simulink model "LQR_control"  (R2025b)
settings: Solver=VariableStepAuto  StartTime=0.0  StopTime=10.0  RelTol=1e-3
values from neighbouring files (symbols this model uses):
  A_Mat = [ 0     1    0     0 ... (first row only)    [LQR_code.m]
  B_Mat = [ 0 ... (first row only)    [LQR_code.m]
  C_Mat = [ 1  0    0   0 ... (first row only)    [LQR_code.m]
  K = lqr(A_Mat, B_Mat, Q, R)    [LQR_code.m]
settings Model: Creator=Mahmoud Essam  LastModifiedBy=Mahmoud Essam

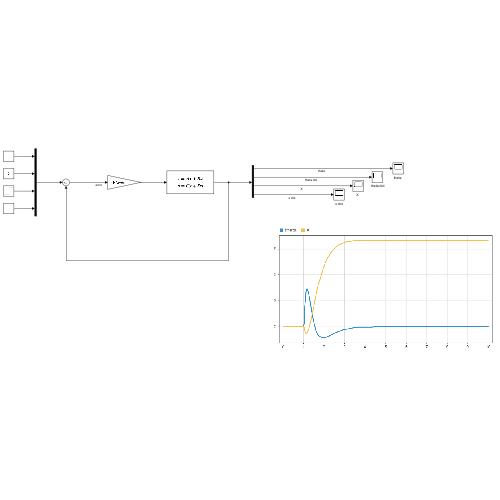
[thumbnail: Simulink's stored preview of the top-level diagram]
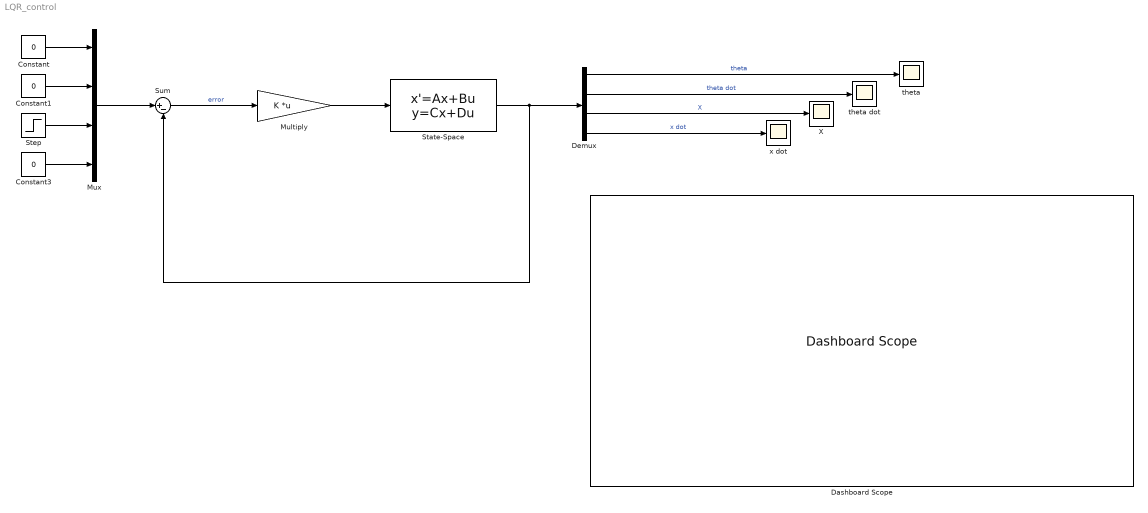
== system LQR_control ==
  " theta dot" : Scope
      settings: ActiveDisplayYMinimum=-22.999413149940512  ActiveDisplayYMaximum=55.548140907039681
  Constant : Constant  Value=0
  Constant1 : Constant  Value=0
  Constant3 : Constant  Value=0
  Dashboard Scope : DashboardScope  FontColor=[0.0, 0.0, 0.0]
  Demux : Demux
  Multiply : Gain  Gain=K  Multiplication=Matrix(K*u) (u vector)
  Mux : Mux
  State-Space : StateSpace  A=A_Mat  B=B_Mat  C=C_Mat  D=[0 ; 0 ; 0; 0]  InitialCondition=0
  Step : Step  After=10  SampleTime=0
  Sum : Sum  Inputs=|+-
  "X " : Scope
      settings: ActiveDisplayYMinimum=-1  ActiveDisplayYMaximum=1  DataLoggingVariableName=ScopeData2
  "theta " : Scope
      settings: ActiveDisplayYMinimum=-1  ActiveDisplayYMaximum=1
  x dot : Scope
      settings: ActiveDisplayYMinimum=-1  ActiveDisplayYMaximum=1  DataLoggingVariableName=ScopeData3
  wires:
  Demux/1 -> "theta "/1  "theta"
  Demux/2 -> " theta dot"/1  "theta dot"
  Multiply/1 -> State-Space/1
  Demux/4 -> x dot/1  "x dot"
  Sum/1 -> Multiply/1  "error"
  State-Space/1 -> Sum/2, Demux/1
  Demux/3 -> "X "/1  "X"
  Mux/1 -> Sum/1
  Constant3/1 -> Mux/4
  Step/1 -> Mux/3
  Constant1/1 -> Mux/2
  Constant/1 -> Mux/1
